simulink model "Clark"  (R2020a)
settings: Solver=VariableStepAuto  StartTime=0.0  StopTime=10.0  RelTol=1e-3
libraries: powerlib_meascontrol x1
settings Model: Creator=Lenovo  LastModifiedBy=Lenovo

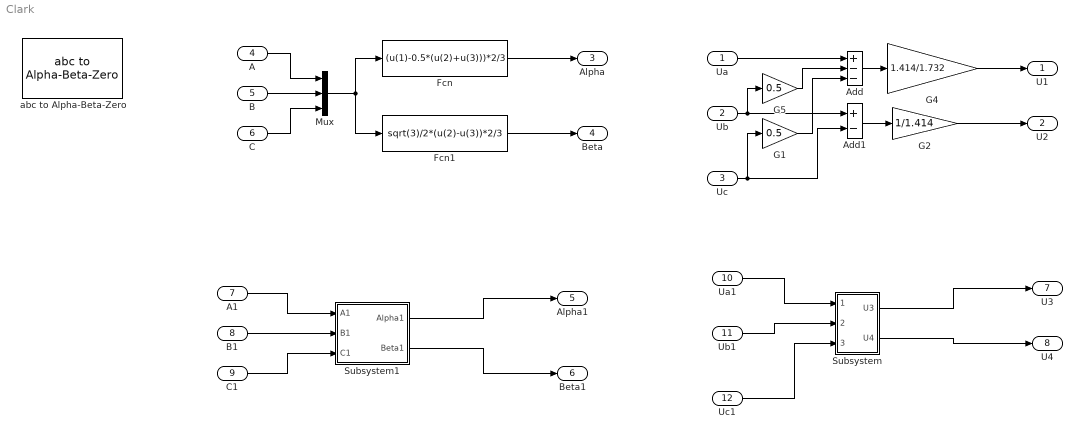
== system Clark ==
  Ua : Inport
  Ub : Inport  Port=2
  Uc : Inport  Port=3
  A : Inport  Port=4
  B : Inport  Port=5
  C : Inport  Port=6
  A1 : Inport  Port=7
  B1 : Inport  Port=8
  C1 : Inport  Port=9
  Ua1 : Inport  Port=10
  Ub1 : Inport  Port=11
  Uc1 : Inport  Port=12
  Add : Sum  Inputs=+--
  Add1 : Sum  Inputs=+-
  Fcn : Fcn  Expr=(u(1)-0.5*(u(2)+u(3)))*2/3
  Fcn1 : Fcn  Expr=sqrt(3)/2*(u(2)-u(3))*2/3
  G1 : Gain  Gain=0.5
  G2 : Gain  Gain=1/1.414
  G4 : Gain  Gain=1.414/1.732
  G5 : Gain  Gain=0.5
  Mux : Mux  Inputs=3
  Subsystem : Subsystem
  Subsystem1 : Subsystem
  abc to Alpha-Beta-Zero : powerlib_meascontrol/Transformations/abc to Alpha-Beta-Zero
  U1 : Outport
  U2 : Outport  Port=2
  Alpha : Outport  Port=3  VectorParamsAs1DForOutWhenUnconnected=off
  Beta : Outport  Port=4  VectorParamsAs1DForOutWhenUnconnected=off
  Alpha1 : Outport  Port=5  VectorParamsAs1DForOutWhenUnconnected=off
  Beta1 : Outport  Port=6  VectorParamsAs1DForOutWhenUnconnected=off
  U3 : Outport  Port=7
  U4 : Outport  Port=8
  wires:
  G4/1 -> U1/1
  G1/1 -> Add/3
  G5/1 -> Add/2
  G2/1 -> U2/1
  Add1/1 -> G2/1
  Uc/1 -> G1/1, Add1/2
  Ua/1 -> Add/1
  Add/1 -> G4/1
  Ub/1 -> G5/1, Add1/1
  Mux/1 -> Fcn1/1, Fcn/1
  Fcn1/1 -> Beta/1
  A/1 -> Mux/1
  Fcn/1 -> Alpha/1
  C/1 -> Mux/3
  B/1 -> Mux/2
  Ua1/1 -> Subsystem/1(Ua1)
  Ub1/1 -> Subsystem/2(Ub1)
  Uc1/1 -> Subsystem/3(Uc1)
  Subsystem/1(U3) -> U3/1
  Subsystem/2(U4) -> U4/1
  A1/1 -> Subsystem1/1(A1)
  B1/1 -> Subsystem1/2(B1)
  C1/1 -> Subsystem1/3(C1)
  Subsystem1/1(Alpha1) -> Alpha1/1
  Subsystem1/2(Beta1) -> Beta1/1

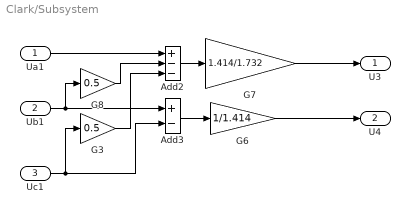
== system Clark/Subsystem ==
  Ua1 : Inport
  Ub1 : Inport  Port=2
  Uc1 : Inport  Port=3
  Add2 : Sum  Inputs=+--
  Add3 : Sum  Inputs=+-
  G3 : Gain  Gain=0.5
  G6 : Gain  Gain=1/1.414
  G7 : Gain  Gain=1.414/1.732
  G8 : Gain  Gain=0.5
  U3 : Outport
  U4 : Outport  Port=2
  wires:
  G3/1 -> Add2/3
  G8/1 -> Add2/2
  Ub1/1 -> G8/1, Add3/1
  Uc1/1 -> G3/1, Add3/2
  Add2/1 -> G7/1
  G6/1 -> U4/1
  Add3/1 -> G6/1
  G7/1 -> U3/1
  Ua1/1 -> Add2/1

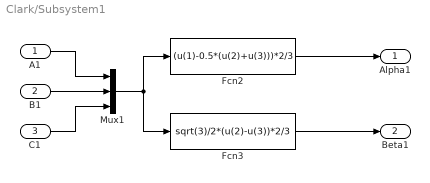
== system Clark/Subsystem1 ==
  A1 : Inport
  B1 : Inport  Port=2
  C1 : Inport  Port=3
  Fcn2 : Fcn  Expr=(u(1)-0.5*(u(2)+u(3)))*2/3
  Fcn3 : Fcn  Expr=sqrt(3)/2*(u(2)-u(3))*2/3
  Mux1 : Mux  Inputs=3
  Alpha1 : Outport  VectorParamsAs1DForOutWhenUnconnected=off
  Beta1 : Outport  Port=2  VectorParamsAs1DForOutWhenUnconnected=off
  wires:
  Mux1/1 -> Fcn3/1, Fcn2/1
  A1/1 -> Mux1/1
  C1/1 -> Mux1/3
  Fcn3/1 -> Beta1/1
  B1/1 -> Mux1/2
  Fcn2/1 -> Alpha1/1
